simulink model "l5"  (R2024a)
settings: Solver=FixedStepAuto  StartTime=0.0  StopTime=inf  RelTol=1e-3
libraries: robotlib x5
settings Model: Creator=ZY395  LastModifiedBy=ZY395
settings OptimizationCC: EnhancedBackFolding=on  PassReuseOutputArgsAs=Individual arguments  ZeroExternalMemoryAtStartup=off  ZeroInternalMemoryAtStartup=off  MaxStackSize=64  OptimizeBlockOrder=speed  DifferentSizesBufferReuse=on  OptimizationCustomize=off  EfficientTunableParamExpr=on
settings DebuggingCC: ParameterTunabilityLossMsg=error
settings HardwareCC: ProdBitPerPointer=32  ProdBitPerSizeT=32  ProdBitPerPtrDiffT=32  ProdLargestAtomicFloat=None  ProdIntDivRoundTo=Undefined  ProdEndianess=Unspecified  ProdWordSize=32  ProdHWDeviceType=Generic->Unspecified (assume 32-bit Generic)
settings SFSimCC: MATLABDynamicMemAlloc=off
settings RTWCC: Description=Embedded Coder  SystemTargetFile=ert.tlc  HardwareBoard=Robot Operating System (ROS)  TLCOptions="-aInlineSetEventsForThisBaseRateFcn=TLC_FALSE -aSuppressMultiTaskScheduler=TLC_FALSE  -aRateBasedStepFcn=0"  TemplateMakefile=ert_default_tmf  Toolchain=Catkin  TargetLang=C++
settings CodeAppCC: ForceParamTrailComments=on  IgnoreCustomStorageClasses=off  OperatorAnnotations=on  SimulinkDataObjDesc=on  SFDataObjDesc=on  InsertBlockDesc=on
settings ERTTargetCC: SupportContinuousTime=on  SupportNonInlinedSFcns=on

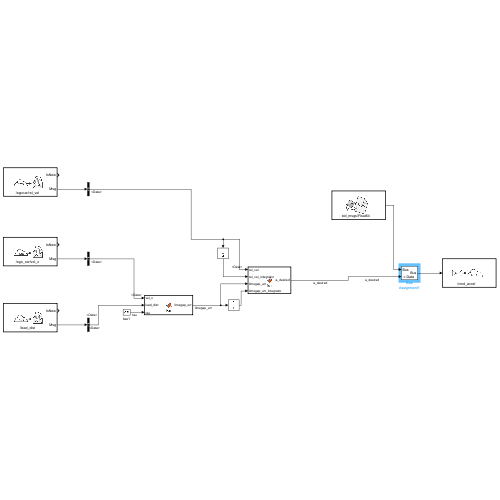
[thumbnail: Simulink's stored preview of the top-level diagram]
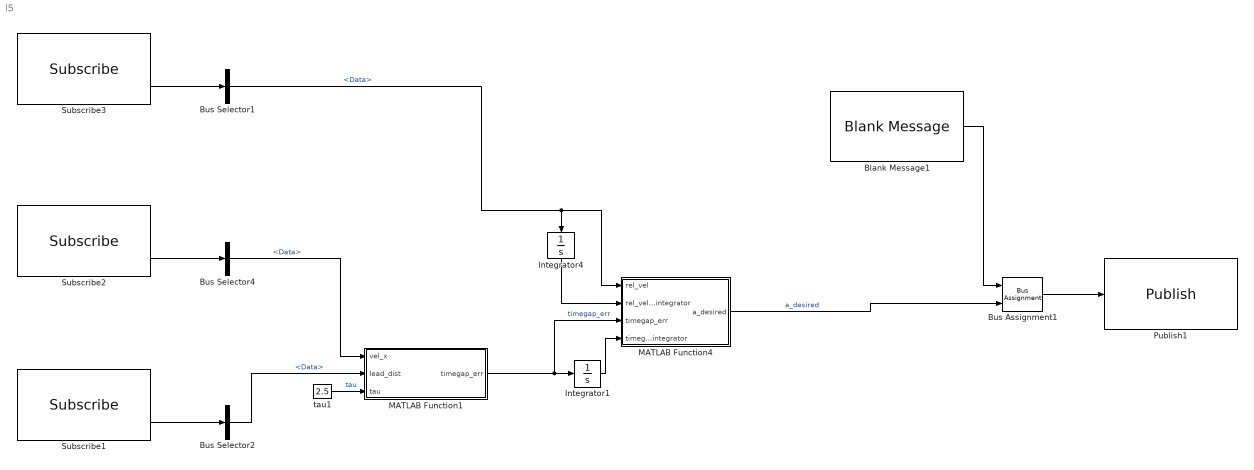
== system l5 ==
  Blank Message1 : robotlib/Blank Message  messageClass=Message  entityType=std_msgs/Float64  messageType=std_msgs/Float64  SampleTime=inf  legacyBusStruct=off
  Bus Assignment1 : BusAssignment  AssignedSignals=Data
  Bus Selector1 : BusSelector  OutputSignals=Data
  Bus Selector2 : BusSelector  OutputSignals=Data
  Bus Selector4 : BusSelector  OutputSignals=Data
  Integrator1 : Integrator
  Integrator4 : Integrator
  MATLAB Function1 : MATLAB Function  TreatAsAtomicUnit=on
  MATLAB Function4 : MATLAB Function  TreatAsAtomicUnit=on
  Publish1 : robotlib/Publish  topicSource=Specify your own  topic=/cmd_accel  messageType=std_msgs/Float64  legacyBusStruct=off  messageQueueLength=1
  Subscribe1 : robotlib/Subscribe  topicSource=Specify your own  topic=/lead_dist  messageType=std_msgs/Float64  SampleTime=-1  legacyBusStruct=off  messageQueueLength=1
  Subscribe2 : robotlib/Subscribe  topicSource=Specify your own  topic=/ego_car/vel_x  messageType=std_msgs/Float64  SampleTime=-1  legacyBusStruct=off  messageQueueLength=1
  Subscribe3 : robotlib/Subscribe  topicSource=Specify your own  topic=/egocar/rel_vel  messageType=std_msgs/Float64  SampleTime=-1  legacyBusStruct=off  messageQueueLength=1
  tau1 : Constant  Value=2.5
  wires:
  Blank Message1/1 -> Bus Assignment1/1
  Bus Assignment1/1 -> Publish1/1
  Bus Selector2/1 -> MATLAB Function1/2(lead_dist)  "<Data>"
  Subscribe1/2 -> Bus Selector2/1
  Subscribe2/2 -> Bus Selector4/1
  Bus Selector4/1 -> MATLAB Function1/1(vel_x)  "<Data>"
  Bus Selector1/1 -> MATLAB Function4/1(rel_vel), Integrator4/1  "<Data>"
  MATLAB Function4/1(a_desired) -> Bus Assignment1/2  "a_desired"
  Subscribe3/2 -> Bus Selector1/1
  tau1/1 -> MATLAB Function1/3(tau)  "tau"
  Integrator1/1 -> MATLAB Function4/4(timegap_err_integrator)
  MATLAB Function1/1(timegap_err) -> MATLAB Function4/3(timegap_err), Integrator1/1  "timegap_err"
  Integrator4/1 -> MATLAB Function4/2(rel_vel_integrator)

== matlab function l5/MATLAB Function1 ==
  data: vel_x input; lead_dist input; tau input; timegap_err output
function timegap_err = fcn(vel_x, lead_dist, tau)

timegap_err = (lead_dist-1)/tau - vel_x; % keep at least 1 meter as safety distance even if both vehicles stop

== matlab function l5/MATLAB Function4 ==
  data: rel_vel input; rel_vel_integrator input; a_desired output; timegap_err input; timegap_err_integrator input
function a_desired = fcn(rel_vel, rel_vel_integrator, timegap_err, timegap_err_integrator)
%delt_tau = 0.5;
%tau_max = tau+delt_tau;
%tau_min = tau-delt_tau;
%time_gap = lead_dist/vel_x;

%if time_gap<tau_max && time_gap>tau_min && rel_vel<2
%    ratio = abs(time_gap-timegap_err)/delt_tau;
%    a=a*(exp(ratio)-1)/(exp(1)-1);
%end

alpha1 = 0.8
alpha2 = .5

a = alpha1*rel_vel + alpha2*timegap_err;

%if rel_vel>0 && a<0
%    a = a + 0.001*timegap_err_integrator + 0.001*rel_vel_integrator;
%end

if rel_vel<0 && a>0
    a=0.01*a
end

maxa=1.5;
mina=-3;
a = min(max(mina,a), maxa);


a_desired = a;
